simulink model "slave_exec"  (Simulink 3.00)
libraries: execlib x6

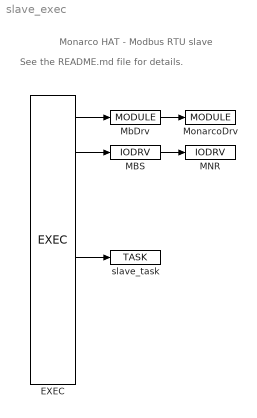
== system slave_exec ==
  note: See the README.md file for details.
  note: Monarco HAT - Modbus RTU slave
  EXEC : execlib/EXEC  target=Generic target device  tick=0.05  ntick0=1  ntick1=20  ntick2=100  ntick3=1200  pri0=5  pri1=9  pri2=13  pri3=18
  MBS : execlib/IODRV  module=MbDrv  classname=MbsDrv  cfgname=slave_cfg.rio  factor=1  stack=10240  pri=3  timer=off
  MNR : execlib/IODRV  module=MonarcoDrv  classname=MonarcoHatDrv  cfgname=monarco.rio  factor=1  stack=10240  pri=3  timer=off
  MbDrv : execlib/MODULE
  MonarcoDrv : execlib/MODULE
  slave_task : execlib/TASK  factor=1  start=0  stop=1  stack=10240  MDLOPEN=on
  wires:
  EXEC/1 -> MbDrv/1
  EXEC/2 -> MBS/1
  EXEC/5 -> slave_task/1
  MBS/1 -> MNR/1
  MbDrv/1 -> MonarcoDrv/1
